simulink model "q6_simulink_modeltotalnonlinearsystem"  (R2024b)
settings: Solver=VariableStepAuto  StartTime=0.0  StopTime=300  RelTol=1e-3
settings Model: Creator=smrut  LastModifiedBy=smrut

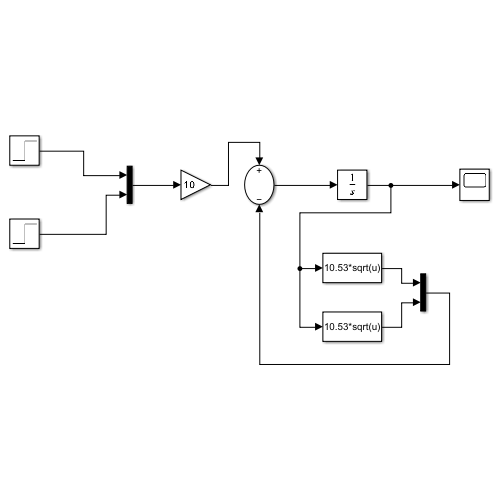
[thumbnail: Simulink's stored preview of the top-level diagram]
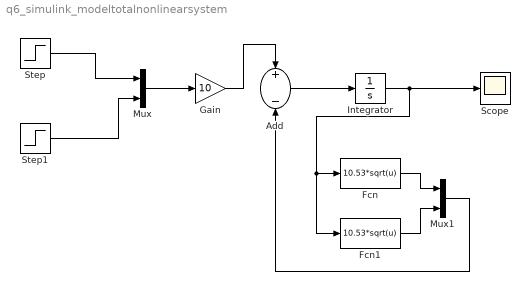
== system q6_simulink_modeltotalnonlinearsystem ==
  Add : Sum  Inputs=+-
  Fcn : Fcn  Expr=10.53*sqrt(u)
  Fcn1 : Fcn  Expr=10.53*sqrt(u)
  Gain : Gain  Gain=10
  Integrator : Integrator  InitialCondition=14
  Mux : Mux  Inputs=2
  Mux1 : Mux  Inputs=2
  Scope : Scope
  Step : Step  Time=0  SampleTime=0
  Step1 : Step  Time=0  SampleTime=0
  wires:
  Step/1 -> Mux/1
  Step1/1 -> Mux/2
  Mux/1 -> Gain/1
  Gain/1 -> Add/1
  Add/1 -> Integrator/1
  Integrator/1 -> Scope/1, Fcn1/1, Fcn/1
  Fcn/1 -> Mux1/1
  Fcn1/1 -> Mux1/2
  Mux1/1 -> Add/2
